simulink model "atrias_gear_dynamics"  (R2017a)
settings: Solver=ode45  StartTime=0.0  StopTime=sim_t  RelTol=1e-3  EnableMultiTasking=on
values from neighbouring files (symbols this model uses):
  N = grid_slice*1000    [createGrid.m]
  nm = fn_set_vnmc_params(sm, sample_time)    [kernel_scores_NM_mismatch.m]    (also in main_ATRIAS_cluster.m)
  nmc_BLCtrlPar = nmc.BLCtrlPar    [kernel_scores_NM_mismatch.m]    (also in main_ATRIAS_cluster.m)
  nmc_FPCtrlPar = nmc.FPCtrlPar    [kernel_scores_NM_mismatch.m]    (also in main_ATRIAS_cluster.m)
  nmc_LLCtrlPar = nmc.LLCtrlPar    [kernel_scores_NM_mismatch.m]    (also in main_ATRIAS_cluster.m)
  nmc_StCtrlPar = nmc.StCtrlPar    [kernel_scores_NM_mismatch.m]    (also in main_ATRIAS_cluster.m)
  nmc_SwCtrlPar = nmc.SwCtrlPar    [kernel_scores_NM_mismatch.m]    (also in main_ATRIAS_cluster.m)
  nmc_TrCtrlPar = nmc.TrCtrlPar    [kernel_scores_NM_mismatch.m]    (also in main_ATRIAS_cluster.m)
  nStep_switchCtrl = 10    [main_ATRIAS_cluster.m]
  nStep_thr = 1000    [createSimInitial.m]    (also in main_ATRIAS_cluster.m)
  rc_CtrlPar = [rc.k_placement, rc.T_step, rc.Cd, rc.kpt, rc.kdt, rc.desired_theta, rc.desired_z, rc.kpz, rc.kdz]    [kernel_scores_NM_mismatch.m]    (also in main_ATRIAS_cluster.m)
  sm = fn_set_MechParams(sm)    [kernel_scores_NM_mismatch.m]    (also in main_ATRIAS_cluster.m = fn_set_MechParams(sm,perturb))
  test_VNMC = 1    [createSimInitial.m]    (also in main_ATRIAS_cluster.m = 0)
undefined symbols (not defined in the file or in its folder): delta_phi_max, delta_phi_max_buffer, delta_phi_min, DiscIntNeverNeededParam, Discrete, idc, initial_dx_estimate, initial_dy_estimate, initial_dz_estimate, initial_z_estimate, kd_shin_max, kd_shin_min, kd_splay_max, kd_splay_min, kd_thigh_max, kd_thigh_min, kp_shin_max, kp_shin_min, kp_splay_max, kp_splay_min, kp_thigh_max, kp_thigh_min, mc, min_splay_angle, min_splay_buffer, phi_shin_max, phi_shin_max_buffer, phi_shin_min, phi_shin_min_buffer, phi_thigh_max, phi_thigh_max_buffer, phi_thigh_min, phi_thigh_min_buffer, rad, rc, s, sample_time, sgn, sim_d, t_friction, Time, X, Y, Z
libraries: sm_lib x206, nesl_utility x132, simulink x77, simulink_extras x24, mblibv1 x4, ctrlSharedLib x4, commnoisgen2 x1, dspswit3 x1
(part 17 of 17)

== stateflow chart atrias_gear_dynamics/control/Robot-to-NMM Interface/Contact State Machine1/State Machine ==
  state TouchDown
  state Unloading
  state Takeoff
  state Flight
  (junction 91) -> TouchDown
  TouchDown -> (junction 130) [order 2] : [vertical_grf < mc.contact_threshold]
  (junction 93) -> (junction 91)
  (junction 130) -> (junction 128)
  TouchDown -> Unloading [order 1] : [vertical_grf > mc.loaded_threshold]
  Unloading -> Takeoff : [vertical_grf < mc.contact_threshold]
  Takeoff -> Flight : after(rc.t_flight,sec)
  (default) -> Flight
  Flight -> (junction 93) : [vertical_grf > mc.contact_threshold]
  (junction 128) -> Flight
  data: z_velocity input; previous_z_velocity input; vertical_grf input; rc parameter; sm parameter; mc parameter; TouchDown output boolean; Unloading output boolean; Takeoff output boolean; Flight output boolean; vertical_acceleration input

== matlab function atrias_gear_dynamics/ATRIAS_sim/Mechanical System Layer/R Leg/Shin SEA/Rotor and Gearing Virtual approximate/gear dynamics approximate ==
  data: torque_rotor input; torque_load input; mc parameter; phi_l_dd output; phi_r_dd output; torque_torso output; gear_acc output; rotor_acc output
function [phi_l_dd, phi_r_dd, torque_torso, gear_acc, rotor_acc] = gear_dynamics_approx(torque_rotor, torque_load, mc)

% theta is the torso angle
% phi_r is the rotor local angle
% phi_l is the load local angle

N = mc.LEG_MTR_GEAR_RATIO;
It = mc.i_robot;
% It = It(2);
Ir = mc.j_rotor;
Il = mc.j_leg/N;

invM = [1/It 0 ; 0 1/(Ir*N^2)];
tau = [torque_rotor ; torque_load];
K = [-1 1 ; N 1];

out = invM*K*tau;

theta_dd = out(1);
torque_torso = It*theta_dd;

phi_l_dd = out(2) - out(1);
gear_acc = phi_l_dd;
phi_r_dd = N*phi_l_dd; 
rotor_acc = phi_r_dd;

% err = ((N-1)/It)*torque_rotor + (1/(N^2*Ir)+(N-1)^2/(N^2*It))*torque_load - out(2);

== matlab function atrias_gear_dynamics/ATRIAS_sim/Mechanical System Layer/R Leg/Thigh SEA/Rotor and Gearing Virtual approximate/gear dynamics approximate ==
  data: torque_rotor input; torque_load input; mc parameter; phi_l_dd output; phi_r_dd output; torque_torso output; gear_acc output; rotor_acc output
function [phi_l_dd, phi_r_dd, torque_torso, gear_acc, rotor_acc] = gear_dynamics_approx(torque_rotor, torque_load, mc)

% theta is the torso angle
% phi_r is the rotor local angle
% phi_l is the load local angle

N = mc.LEG_MTR_GEAR_RATIO;
It = mc.i_robot;
% It = It(2);
Ir = mc.j_rotor;
Il = mc.j_leg/N;

invM = [1/It 0 ; 0 1/(Ir*N^2)];
tau = [torque_rotor ; torque_load];
K = [-1 1 ; N 1];

out = invM*K*tau;

theta_dd = out(1);
torque_torso = It*theta_dd;

phi_l_dd = out(2) - out(1);
gear_acc = phi_l_dd;
phi_r_dd = N*phi_l_dd; 
rotor_acc = phi_r_dd;

% err = ((N-1)/It)*torque_rotor + (1/(N^2*Ir)+(N-1)^2/(N^2*It))*torque_load - out(2);

== matlab function atrias_gear_dynamics/ATRIAS_sim/Mechanical System Layer/Torso/Rotation To Euler Angles ==
  data: R input; roll output; pitch output; yaw output
function  [roll, pitch, yaw] = rotation_to_euler(R)  
    
    persistent curyaw
    if isempty(curyaw)
        curyaw = 0;
    end

    newyaw = atan2( R(2,1), R(1,1));
    pitch  = atan2(-R(3,1), sqrt(R(3,2)^2+R(3,3)^2));
    roll   = atan2( R(3,2), R(3,3));
    curyaw = curyaw + mod(newyaw - curyaw + pi, 2*pi) - pi;
    yaw = curyaw;
    
end

== matlab function atrias_gear_dynamics/control/Virtual Neuromuscular Control/Torque Distribution/mech limit avoidance1/PD Joint Limit1/to hip_knee ==
  data: Rtau_back input; tau_pd_hip_knee output; Rtau_front input; Ltau_back input; Ltau_front input; kR input; kL input
function tau_pd_hip_knee = fcn(Rtau_back,Rtau_front,Ltau_back,Ltau_front,kR,kL)

J_inv_trans = [1,1,0,0;
               -((kR+1)/(2*kR)),-((kR-1)/(2*kR)),0,0;
               0,0,1,1;
               0,0,-((kL+1)/(2*kL)),-((kL-1)/(2*kL))];
           
tau_pd_hip_knee = J_inv_trans*[Rtau_back;
                               Rtau_front;
                               Ltau_back;
                               Ltau_front];

== matlab function atrias_gear_dynamics/control/RC control/Inverse Dynamics 2D/target_GRF_inverse_dynamics ==
  data: GRFx input; GRFz input; z output; theta input; phi input; l_leg input; w input; tau_rotor_f input; tau_rotor_b input; mc parameter
%% Inverse dynamics
% Inputs:  gamma, dgamma, theta, dtheta,  GRFx_des, GRFy_des
% Outputs: ddx,   ddy,    ddl,   ddgamma, ddtheta,  tau_sf,  tau_sb
function z = fcn(GRFx, GRFz, theta, phi, l_leg, w,...
                                  tau_rotor_f, tau_rotor_b, ...
                                  mc)
              
    % Parameters
    m      = mc.m_total_real;    % mass of system + boom
    Il     = mc.j_leg;             % inertia of leg
    It     = mc.i_robot;           % inertia of system3.
    d      = mc.d_vertical_com;             % distance from hip to system COM
    g1     = phi(1)+theta(1);   % global leg angle (after spring)
    dg1    = phi(2)+theta(2);
    th     = theta(1);          % global torso angle   
    dth    = theta(2);
    t_rf   = tau_rotor_f;       % torque applied at front rotor 
    t_rb   = tau_rotor_b;       % torque applied at back rotor
    N      = -mc.LEG_MTR_GEAR_RATIO;
    l      = l_leg(1);          % leg length
    dl     = l_leg(2);
    g = mc.g;
    m_leg = mc.m_leg;
    
    % Stance dynamics (P z = [h; -dJ*dq] + [J zeros(2,2)]^T F)
    %     J  = [1  0  sin(g1)     l*cos(g1)   -d*cos(th);
    %           0  1  cos(g1)    -l*sin(g1)    d*sin(th)];
    %       
    %     dJ = [0  0   dg1*cos(g1)    (-l*dg1*sin(g1)+dl*cos(g1))  d*dth*sin(th);
    %           0  0  -dg1*sin(g1)    (-1*dg1*cos(g1)-dl*sin(g1))  d*dth*cos(th)];
    % 
    %     dq  = [dx  dz  dl  dg1  dth ]';
    %       
    %     M = [m  0   0       0    0; 
    %          0  m   0       0    0;
    %          0  0   m_leg   0    0;   
    %          0  0   0       Il   0;  
    %          0  0   0       0    It];  
    %     
    %     h = [0; -m*g_reduced; 0; 0; (-t_rf-t_rb)];
    % 
    %     S = [ 0         0;
    %           0         0;
    %           1/w      -1/w;
    %           1         1;
    %          -(N-1)/N  -(N-1)/N];
    % 
    %     F = [GRFx GRFz]';
    %     
    %     P = [M              -S;       
    %          J               zeros(2,2)];
    
    % Solving for z:    
    %     ddq = [ddx ddy ddl ddg1 ddth]';
    %     z = [ddq; t_sf; t_sb];
    %     z = P\([h; -dJ*dq] + [J zeros(2,2)]'*F);
    
    z =  [GRFx/m;
         (GRFz - g*m)/m;
        -(Il*d*dg1^2*m*cos(g1 - th) - 2*GRFx*Il*d*sin(th) - 2*Il*d^2*dth^2*m - GRFz*d*l^2*m*cos(th) - GRFx*d*l^2*m*sin(th) - 2*GRFz*Il*d*cos(th) + 2*GRFz*It*N*l*cos(g1) + 2*GRFz*Il*N*d*cos(th) + 2*GRFx*It*N*l*sin(g1) + 2*GRFx*Il*N*d*sin(th) - It*N*dg1^2*l*m + GRFz*d*l^2*m*cos(2*g1 - th) + GRFx*d*l^2*m*sin(2*g1 - th) + 2*Il*d*g*m*cos(th) + Il*d*dg1^2*m*cos(g1 + th) + 2*Il*N*d^2*dth^2*m - It*N*dg1^2*l^2*m - 2*It*N*g*l*m*cos(g1) - 2*Il*N*d*g*m*cos(th) + It*N*dg1^2*l^2*m*cos(2*g1) - Il*N*d*dg1^2*m*cos(g1 + th) - Il*d*dg1^2*l*m*cos(g1 + th) + 4*Il*d*dg1*dl*m*sin(g1 - th) + GRFz*N*d^2*l*m*cos(g1) + GRFz*N*d*l^2*m*cos(th) + GRFx*N*d^2*l*m*sin(g1) + 2*N*d*l*m*t_rb*sin(g1 - th) + 2*N*d*l*m*t_rf*sin(g1 - th) + GRFx*N*d*l^2*m*sin(th) - Il*N*d*dg1^2*m*cos(g1 - th) - GRFz*N*d^2*l*m*cos(g1 - 2*th) + GRFx*N*d^2*l*m*sin(g1 - 2*th) + Il*d*dg1^2*l*m*cos(g1 - th) - It*N*dg1^2*l*m*cos(2*g1) - GRFz*N*d*l^2*m*cos(2*g1 - th) - GRFx*N*d*l^2*m*sin(2*g1 - th) + Il*N*d*dg1^2*l*m*cos(g1 + th) - 4*Il*N*d*dg1*dl*m*sin(g1 - th) - Il*N*d*dg1^2*l*m*cos(g1 - th) + 2*It*N*d*dth^2*l*m*cos(g1 - th))/(2*m*(It*N*l - Il*d*cos(g1 - th) + Il*N*d*cos(g1 - th)));
        -(2*GRFx*It*N*cos(g1) - 2*GRFz*It*N*sin(g1) + GRFx*N*d^2*m*cos(g1 - 2*th) + 4*It*N*dg1*dl*m + GRFz*N*d^2*m*sin(g1 - 2*th) + GRFx*d*l*m*cos(2*g1 - th) - GRFz*d*l*m*sin(2*g1 - th) + It*N*dg1^2*m*sin(2*g1) + 2*It*N*g*m*sin(g1) + GRFx*d*l*m*cos(th) - GRFz*d*l*m*sin(th) + GRFx*N*d^2*m*cos(g1) + 2*N*d*m*t_rb*cos(g1 - th) + 2*N*d*m*t_rf*cos(g1 - th) - GRFz*N*d^2*m*sin(g1) - GRFx*N*d*l*m*cos(th) + GRFz*N*d*l*m*sin(th) - GRFx*N*d*l*m*cos(2*g1 - th) - 2*It*N*d*dth^2*m*sin(g1 - th) + GRFz*N*d*l*m*sin(2*g1 - th) - It*N*dg1^2*l*m*sin(2*g1))/(2*m*(It*N*l - Il*d*cos(g1 - th) + Il*N*d*cos(g1 - th)));
        -(GRFx*Il*cos(g1) - GRFz*Il*sin(g1) - GRFx*Il*N*cos(g1) + (Il*dg1^2*m*sin(2*g1))/2 + GRFz*Il*N*sin(g1) + Il*g*m*sin(g1) + GRFx*l^2*m*cos(g1) - GRFz*l^2*m*sin(g1) + 2*Il*dg1*dl*m + N*l*m*t_rb + N*l*m*t_rf + GRFz*N*l^2*m*sin(g1) - 2*Il*N*dg1*dl*m - Il*d*dth^2*m*sin(g1 - th) - (Il*N*dg1^2*m*sin(2*g1))/2 - (Il*dg1^2*l*m*sin(2*g1))/2 - Il*N*g*m*sin(g1) - GRFx*N*l^2*m*cos(g1) + GRFx*N*d*l*m*cos(th) - GRFz*N*d*l*m*sin(th) + Il*N*d*dth^2*m*sin(g1 - th) + (Il*N*dg1^2*l*m*sin(2*g1))/2)/(m*(It*N*l - Il*d*cos(g1 - th) + Il*N*d*cos(g1 - th)));
        -(2*GRFx*Il*It*N*cos(g1) - 2*GRFz*Il*It*N*sin(g1) - GRFz*Il*d*m*w*cos(th) - 2*GRFz*Il*d*m_leg*w*cos(th) - GRFx*Il*d*m*w*sin(th) - 2*GRFx*Il*d*m_leg*w*sin(th) + GRFx*Il*N*d^2*m*cos(g1) + 2*Il*N*d*m*t_rb*cos(g1 - th) + 2*Il*N*d*m*t_rf*cos(g1 - th) + 2*GRFx*It*N*l^2*m*cos(g1) - GRFz*Il*N*d^2*m*sin(g1) - 2*GRFz*It*N*l^2*m*sin(g1) + GRFx*Il*N*d^2*m*cos(g1 - 2*th) + 4*Il*It*N*dg1*dl*m + GRFz*Il*N*d^2*m*sin(g1 - 2*th) - 2*Il*d^2*dth^2*m*m_leg*w - GRFz*Il*d*m*w*cos(2*g1 - th) - GRFx*Il*d*m*w*sin(2*g1 - th) + Il*It*N*dg1^2*m*sin(2*g1) + 2*Il*It*N*g*m*sin(g1) - GRFx*d*l^2*m*m_leg*w*sin(th) - Il*It*N*dg1^2*l*m*sin(2*g1) + Il*d*dg1^2*m*m_leg*w*cos(g1 - th) + 2*GRFz*It*N*l*m*w*cos(g1) + 2*GRFz*It*N*l*m_leg*w*cos(g1) + GRFz*Il*N*d*m*w*cos(th) + 2*GRFz*Il*N*d*m_leg*w*cos(th) + 2*GRFx*It*N*l*m*w*sin(g1) + 2*GRFx*It*N*l*m_leg*w*sin(g1) + GRFx*Il*N*d*m*w*sin(th) + 2*GRFx*Il*N*d*m_leg*w*sin(th) - It*N*dg1^2*l*m*m_leg*w + GRFz*d*l^2*m*m_leg*w*cos(2*g1 - th) + GRFx*d*l^2*m*m_leg*w*sin(2*g1 - th) + 2*Il*d*g*m*m_leg*w*cos(th) + Il*d*dg1^2*m*m_leg*w*cos(g1 + th) + 2*Il*N*d^2*dth^2*m*m_leg*w - It*N*dg1^2*l^2*m*m_leg*w - 2*Il*It*N*d*dth^2*m*sin(g1 - th) + GRFz*Il*N*d*m*w*cos(2*g1 - th) + GRFx*Il*N*d*m*w*sin(2*g1 - th) - GRFz*d*l^2*m*m_leg*w*cos(th) + It*N*dg1^2*l^2*m*m_leg*w*cos(2*g1) - Il*N*d*dg1^2*m*m_leg*w*cos(g1 + th) - Il*d*dg1^2*l*m*m_leg*w*cos(g1 + th) + 4*Il*d*dg1*dl*m*m_leg*w*sin(g1 - th) + GRFz*N*d^2*l*m*m_leg*w*cos(g1) + GRFz*N*d*l^2*m*m_leg*w*cos(th) + GRFx*N*d^2*l*m*m_leg*w*sin(g1) + 2*N*d*l*m*m_leg*t_rb*w*sin(g1 - th) + 2*N*d*l*m*m_leg*t_rf*w*sin(g1 - th) + GRFx*N*d*l^2*m*m_leg*w*sin(th) - Il*N*d*dg1^2*m*m_leg*w*cos(g1 - th) - GRFz*N*d^2*l*m*m_leg*w*cos(g1 - 2*th) + GRFx*N*d^2*l*m*m_leg*w*sin(g1 - 2*th) + Il*d*dg1^2*l*m*m_leg*w*cos(g1 - th) - It*N*dg1^2*l*m*m_leg*w*cos(2*g1) - GRFz*N*d*l^2*m*m_leg*w*cos(2*g1 - th) - GRFx*N*d*l^2*m*m_leg*w*sin(2*g1 - th) - 2*It*N*g*l*m*m_leg*w*cos(g1) - 2*Il*N*d*g*m*m_leg*w*cos(th) + Il*N*d*dg1^2*l*m*m_leg*w*cos(g1 + th) - 4*Il*N*d*dg1*dl*m*m_leg*w*sin(g1 - th) - Il*N*d*dg1^2*l*m*m_leg*w*cos(g1 - th) + 2*It*N*d*dth^2*l*m*m_leg*w*cos(g1 - th))/(4*m*(It*N*l - Il*d*cos(g1 - th) + Il*N*d*cos(g1 - th)));
         (2*GRFz*Il*It*N*sin(g1) - 2*GRFx*Il*It*N*cos(g1) - GRFz*Il*d*m*w*cos(th) - 2*GRFz*Il*d*m_leg*w*cos(th) - GRFx*Il*d*m*w*sin(th) - 2*GRFx*Il*d*m_leg*w*sin(th) - GRFx*Il*N*d^2*m*cos(g1) - 2*Il*N*d*m*t_rb*cos(g1 - th) - 2*Il*N*d*m*t_rf*cos(g1 - th) - 2*GRFx*It*N*l^2*m*cos(g1) + GRFz*Il*N*d^2*m*sin(g1) + 2*GRFz*It*N*l^2*m*sin(g1) - GRFx*Il*N*d^2*m*cos(g1 - 2*th) - 4*Il*It*N*dg1*dl*m - GRFz*Il*N*d^2*m*sin(g1 - 2*th) - 2*Il*d^2*dth^2*m*m_leg*w - GRFz*Il*d*m*w*cos(2*g1 - th) - GRFx*Il*d*m*w*sin(2*g1 - th) - Il*It*N*dg1^2*m*sin(2*g1) - 2*Il*It*N*g*m*sin(g1) - GRFx*d*l^2*m*m_leg*w*sin(th) + Il*It*N*dg1^2*l*m*sin(2*g1) + Il*d*dg1^2*m*m_leg*w*cos(g1 - th) + 2*GRFz*It*N*l*m*w*cos(g1) + 2*GRFz*It*N*l*m_leg*w*cos(g1) + GRFz*Il*N*d*m*w*cos(th) + 2*GRFz*Il*N*d*m_leg*w*cos(th) + 2*GRFx*It*N*l*m*w*sin(g1) + 2*GRFx*It*N*l*m_leg*w*sin(g1) + GRFx*Il*N*d*m*w*sin(th) + 2*GRFx*Il*N*d*m_leg*w*sin(th) - It*N*dg1^2*l*m*m_leg*w + GRFz*d*l^2*m*m_leg*w*cos(2*g1 - th) + GRFx*d*l^2*m*m_leg*w*sin(2*g1 - th) + 2*Il*d*g*m*m_leg*w*cos(th) + Il*d*dg1^2*m*m_leg*w*cos(g1 + th) + 2*Il*N*d^2*dth^2*m*m_leg*w - It*N*dg1^2*l^2*m*m_leg*w + 2*Il*It*N*d*dth^2*m*sin(g1 - th) + GRFz*Il*N*d*m*w*cos(2*g1 - th) + GRFx*Il*N*d*m*w*sin(2*g1 - th) - GRFz*d*l^2*m*m_leg*w*cos(th) + It*N*dg1^2*l^2*m*m_leg*w*cos(2*g1) - Il*N*d*dg1^2*m*m_leg*w*cos(g1 + th) - Il*d*dg1^2*l*m*m_leg*w*cos(g1 + th) + 4*Il*d*dg1*dl*m*m_leg*w*sin(g1 - th) + GRFz*N*d^2*l*m*m_leg*w*cos(g1) + GRFz*N*d*l^2*m*m_leg*w*cos(th) + GRFx*N*d^2*l*m*m_leg*w*sin(g1) + 2*N*d*l*m*m_leg*t_rb*w*sin(g1 - th) + 2*N*d*l*m*m_leg*t_rf*w*sin(g1 - th) + GRFx*N*d*l^2*m*m_leg*w*sin(th) - Il*N*d*dg1^2*m*m_leg*w*cos(g1 - th) - GRFz*N*d^2*l*m*m_leg*w*cos(g1 - 2*th) + GRFx*N*d^2*l*m*m_leg*w*sin(g1 - 2*th) + Il*d*dg1^2*l*m*m_leg*w*cos(g1 - th) - It*N*dg1^2*l*m*m_leg*w*cos(2*g1) - GRFz*N*d*l^2*m*m_leg*w*cos(2*g1 - th) - GRFx*N*d*l^2*m*m_leg*w*sin(2*g1 - th) - 2*It*N*g*l*m*m_leg*w*cos(g1) - 2*Il*N*d*g*m*m_leg*w*cos(th) + Il*N*d*dg1^2*l*m*m_leg*w*cos(g1 + th) - 4*Il*N*d*dg1*dl*m*m_leg*w*sin(g1 - th) - Il*N*d*dg1^2*l*m*m_leg*w*cos(g1 - th) + 2*It*N*d*dth^2*l*m*m_leg*w*cos(g1 - th))/(4*m*(It*N*l - Il*d*cos(g1 - th) + Il*N*d*cos(g1 - th)))];


end

== matlab function atrias_gear_dynamics/control/RC control/Primary Secondary Leg Swap/ToggleRightLeftLeg ==
  data: toggle input boolean; right_left output double; previous_right_left input double; time_sim input
function right_left = ToggleRightLeftLeg(toggle, previous_right_left, time_sim)
    
    if toggle && time_sim > 0.1
        right_left = -previous_right_left + 1;
    else
        right_left = previous_right_left;
    end

end

== matlab function atrias_gear_dynamics/control/RC control/Sagittal State Feedback ==
  data: kpt input; kdt input; desired_theta input; Fx output size=1; x_dx input; z_dz input; theta_dtheta input; GRF_z input; idc parameter size=1; rc parameter
function Fx  = sagittal_feedback(kpt, kdt, desired_theta, x_dx, z_dz, theta_dtheta, GRF_z, idc, rc)
    sagittal_state = [x_dx(1),  x_dx(2), theta_dtheta(1), theta_dtheta(2)]';
    sagittal_reference = [0, 0 , desired_theta, 0]';
    sagittal_error = (sagittal_state - sagittal_reference);
    neutral_feedforward = GRF_z*x_dx(1)/z_dz(1);
    Fx_feedback =  -[rc.kpx, rc.kdx, kpt, kdt]*sagittal_error;
    Fx = Fx_feedback + neutral_feedforward;
    Fx = min(max(Fx,-0.5*GRF_z),0.5*GRF_z);
end

== matlab function atrias_gear_dynamics/control/RC control/Swing/swing_trajectory_regenerator ==
  data: T_step input; time_step input size=1; x output size=1; x0 input size=1; xd output size=1; xdd output size=1; z output size=1; zd output size=1; zdd output size=1; nstep input size=1; x1 input size=1; rc parameter size=1
function [x,xd,xdd, z,zd, zdd] = swing_trajectory_generator(T_step, time_step, x0, nstep, x1, rc)

%T_step = rc.T_step;
z_apex = rc.z_apex;

%x0 = -0.2;
dx0= 0.0;
% x1 = x1+0.05;
dx1 = 0.0;
z0 = 0.0;
dz0 = 0.0;
z1 = -0.05;
dz1 = 0.0;
T = T_step;

if(nstep == 1)
%     x0 = 0.0;
%     x1 = 0.2;
    z0 = 0.2;
    dz0 = 0.0;
    T = T_step/2;
end

tf = min(time_step, T);

if(tf < T/2)
    [a0 a1 a2 a3] = ThirdOrderTrajectory(z0, dz0, z_apex, 0.0, T/2);
    t = tf;
    z = a3*t^3 + a2*t^2 + a1*t + a0;
    zd = 3*a3*t^2 + 2*a2*t + a1;
else
    [a0 a1 a2 a3] = ThirdOrderTrajectory(z_apex, 0.0, z1, dz1, T/2);
    t = tf - T/2;
    z = a3*t^3 + a2*t^2 + a1*t + a0;
    zd = 3*a3*t^2 + 2*a2*t + a1;
end

zdd = 0;

[a0 a1 a2 a3] = ThirdOrderTrajectory(x0, dx0, x1, dx1, T);
t = tf;
x = a3*t^3 + a2*t^2 + a1*t + a0;
xd = 3*a3*t^2 + 2*a2*t + a1;
xdd = 6*a3*t + 2*a2;
end

== matlab function atrias_gear_dynamics/control/RC control/Torque Distribution/Motor Torque Saturation Optimization ==
  data: x1s input; t1 output; x2s input; mc parameter; t2 output
% Optimal leg motor torque distribution
function [t1, t2] = distribute_torque(x1s, x2s, mc)

lambda1 = mc.lambda1;
lambda2 = mc.lambda2;
max_torque_sagittal = mc.LEG_MTR_MAX_TORQUE;

s = max_torque_sagittal;

% possible solutions
x1 = [                                                      x1s;
                                                            0;
                                                            s;
                                                            0;
                                                           -s;
  (lambda2*s + lambda1*x1s - lambda2*x2s)/(lambda1 + lambda2);
  (lambda1*x1s - lambda2*s + lambda2*x2s)/(lambda1 + lambda2);
  (lambda2*s + lambda1*x1s + lambda2*x2s)/(lambda1 + lambda2);
 -(lambda2*s - lambda1*x1s + lambda2*x2s)/(lambda1 + lambda2)];
 
x2 = [                                                      x2s;
                                                            s;
                                                            0;
                                                           -s;
                                                            0;
  (lambda1*s - lambda1*x1s + lambda2*x2s)/(lambda1 + lambda2);
  (lambda1*s + lambda1*x1s + lambda2*x2s)/(lambda1 + lambda2);
  (lambda1*x1s - lambda1*s + lambda2*x2s)/(lambda1 + lambda2);
 -(lambda1*s + lambda1*x1s - lambda2*x2s)/(lambda1 + lambda2)];

% test constraints
c1 = s - x1 - x2 >= 0;
c2 = s + x1 + x2 >= 0;
c3 = s - x1 + x2 >= 0;
c4 = s + x1 - x2 >= 0;
constraints = c1 & c2 & c3 & c4;

% objective function to maximize
f = -lambda1*(x1-x1s).^2-lambda2*(x2-x2s).^2;
satisfied = find(constraints);
[~,I] = max(f(satisfied));

t1 = x1(satisfied(I));
t2 = x2(satisfied(I));

== matlab function atrias_gear_dynamics/control/RC control/Compute COM Translational Acceleration (IMU uses non-rotating measurement frame) ==
  data: com_acceleration_world output; torso_angular_accelerations input; imu_translational_accelerations_body input; torso_roll input; torso_pitch input; torso_yaw input; com_position_world input; com_velocity_world input; hip_roll_accelerations input; right_hip_roll input; left_hip_roll input; torso_com_acceleration_world output; pelvis_acceleration_world output; right_hip_acceleration_world output; left_hip_acceleration_world output; com_acceleration_yawed output; mc parameter
function [com_acceleration_world, torso_com_acceleration_world, pelvis_acceleration_world, right_hip_acceleration_world, left_hip_acceleration_world, com_acceleration_yawed] ...
          = compute_com_acceleration(torso_angular_accelerations, imu_translational_accelerations_body, torso_roll, torso_pitch, torso_yaw, ...
          com_position_world, com_velocity_world, ...
          hip_roll_accelerations, right_hip_roll, left_hip_roll, mc)

      pelvis_to_imu = mc.pelvis_to_imu;
      com_torso = mc.com_torso;
      com_leg_motor = mc.com_leg_motor;
      m_leg_motor = mc.m_leg_motor;
      m_leg = mc.m_leg;
      m_torso = mc.m_torso;
      g = mc.g;
      
    % Body frame to Yawed frame rotations  
    R_body_to_yawed = R_pitch(torso_pitch(1))*R_roll(torso_roll(1));
    dR_body_to_yawed = dR_pitch(torso_pitch(1),torso_pitch(2))*R_roll(torso_roll(1)) + R_pitch(torso_pitch(1))*dR_roll(torso_roll(1),torso_roll(2));
    ddR_body_to_yawed = ddR_pitch(torso_pitch(1),torso_pitch(2),torso_angular_accelerations(2))*R_roll(torso_roll(1)) ...
                        + R_pitch(torso_pitch(1))*ddR_roll(torso_roll(1),torso_roll(2),torso_angular_accelerations(1)) ... 
                        + 2*dR_pitch(torso_pitch(1),torso_pitch(2))*dR_roll(torso_roll(1),torso_roll(2));
    % Yawed frame to World frame rotations  
    R_yawed_to_world = R_yaw(torso_yaw(1));
    dR_yawed_to_world = dR_yaw(torso_yaw(1),torso_yaw(2));
    ddR_yawed_to_world = ddR_yaw(torso_yaw(1),torso_yaw(2),torso_angular_accelerations(3));
    % Compute translational acceleration of torso COM
    R_position_body_to_world = R_yawed_to_world*R_body_to_yawed;
    R_velocity_body_to_world = dR_yawed_to_world*R_body_to_yawed + R_yawed_to_world*dR_body_to_yawed;
    R_acceleration_body_to_world = ddR_yawed_to_world*R_body_to_yawed + 2*dR_yawed_to_world*dR_body_to_yawed + R_yawed_to_world*ddR_body_to_yawed;
    imu_to_torso_com_acceleration_world = R_acceleration_body_to_world*(com_torso - pelvis_to_imu)';
    imu_acceleration_world = R_yawed_to_world*R_body_to_yawed*imu_translational_accelerations_body;
    torso_com_acceleration_world = imu_acceleration_world + imu_to_torso_com_acceleration_world;
    % Compute accelerations of hip COMs
    R_right_hip_to_body =     R_roll(-pi/2+right_hip_roll(1));
    dR_right_hip_to_body =   dR_roll(-pi/2+right_hip_roll(1), right_hip_roll(2));
    ddR_right_hip_to_body = ddR_roll(-pi/2+right_hip_roll(1), right_hip_roll(2), hip_roll_accelerations(1));
    R_left_hip_to_body =     R_roll(pi/2-left_hip_roll(1));
    dR_left_hip_to_body =   dR_roll(pi/2-left_hip_roll(1), -left_hip_roll(2));
    ddR_left_hip_to_body = ddR_roll(pi/2-left_hip_roll(1), -left_hip_roll(2), -hip_roll_accelerations(2));
    imu_to_pelvis_com_acceleration_world = R_acceleration_body_to_world*(-pelvis_to_imu)';  
    pelvis_acceleration_world = imu_acceleration_world + imu_to_pelvis_com_acceleration_world;
    left_hip_acceleration_world = pelvis_acceleration_world + (R_acceleration_body_to_world*R_left_hip_to_body + 2*R_velocity_body_to_world*dR_left_hip_to_body + R_position_body_to_world*ddR_left_hip_to_body)*com_leg_motor';
    right_hip_acceleration_world = pelvis_acceleration_world + (R_acceleration_body_to_world*R_right_hip_to_body + 2*R_velocity_body_to_world*dR_right_hip_to_body + R_position_body_to_world*ddR_right_hip_to_body)*(com_leg_motor.*[1,-1,1])';
    % Compute total system COM acceleration
    m_hip = m_leg+m_leg_motor;
    m_total = 2*m_hip + m_torso;
    com_acceleration_world = (m_torso*torso_com_acceleration_world + m_hip*(left_hip_acceleration_world + right_hip_acceleration_world))/m_total;
    com_acceleration_yawed = ddR_yawed_to_world'*com_position_world + 2*dR_yawed_to_world'*com_velocity_world + R_yawed_to_world'*com_acceleration_world;
    com_acceleration_yawed(3) = com_acceleration_yawed(3);% - g;
end

function R_yp = R_pitch(theta) % map from pitched to yawed
  R_yp = [cos(theta), 0, sin(theta); ...
          0, 1, 0; ...
          -sin(theta), 0, cos(theta)];
end
function dR_yp = dR_pitch(theta,dtheta)
  dR_yp = dtheta*[-sin(theta), 0, cos(theta); ...
                  0, 0, 0; ... 
                  -cos(theta), 0, -sin(theta)];
end
function ddR_yp = ddR_pitch(theta,dtheta,ddtheta)
  ddR_yp = ddtheta*[-sin(theta), 0, cos(theta); ...
                    0, 0, 0; ... 
                    -cos(theta), 0, -sin(theta)] ...
           + dtheta^2*[-cos(theta), 0, -sin(theta); ...
                     0, 0, 0; ...
                     sin(theta), 0, -cos(theta)];
end
function R_pr = R_roll(phi) % map from rolled to pitched
  R_pr = [1, 0, 0; ...
          0, cos(phi), -sin(phi); ...
          0, sin(phi), cos(phi)]; 
end
function dR_pr = dR_roll(phi,dphi)
  dR_pr = dphi*[0, 0, 0; ...
                0, -sin(phi), -cos(phi); ...
                0, cos(phi), -sin(phi)];
end
function ddR_pr = ddR_roll(phi, dphi, ddphi)
  ddR_pr = ddphi*[0, 0, 0; ...
                  0, -sin(phi), -cos(phi); ...
                  0, cos(phi), -sin(phi)] ...
           + dphi^2*[0, 0, 0; ...
                   0, -cos(phi), sin(phi);...
                   0, -sin(phi), -cos(phi)];
end
function R_gy = R_yaw(psi) % map yawed frame to global
  R_gy = [cos(psi), -sin(psi), 0; sin(psi), cos(psi), 0; 0 0 1]; 
end
function dR_gy = dR_yaw(psi,dpsi)
  dR_gy = dpsi*[-sin(psi), -cos(psi), 0; cos(psi), -sin(psi), 0; 0 0 0];
end
function ddR_gy = ddR_yaw(psi,dpsi,ddpsi)
  ddR_gy = ddpsi*[-sin(psi), -cos(psi), 0; cos(psi), -sin(psi), 0; 0 0 0] ...
           + dpsi^2*[-cos(psi), sin(psi), 0; -sin(psi), -cos(psi), 0; 0 0 0];
end

== matlab function atrias_gear_dynamics/control/RC control/Compute World Frame COM Coordinates from Yawed Frame ==
  data: com_position_world output; X_dX input; Y_dY input; Z_dZ input; torso_yaw input; com_velocity_world output
function [com_position_world, com_velocity_world] ...
          = compute_com_state_in_world_frame(X_dX, Y_dY, Z_dZ, torso_yaw)

    R_yawed_to_world = R_yaw(torso_yaw(1));
    dR_yawed_to_world = dR_yaw(torso_yaw(1),torso_yaw(2));
    
    com_position_yawed = [X_dX(1); Y_dY(1); Z_dZ(1)];
    com_velocity_yawed = [X_dX(2); Y_dY(2); Z_dZ(2)];
    
    com_position_world = R_yawed_to_world*com_position_yawed;
    com_velocity_world = dR_yawed_to_world*com_position_yawed + R_yawed_to_world*com_velocity_yawed;

end

function R_gy = R_yaw(psi) % map yawed frame to global
  R_gy = [cos(psi), -sin(psi), 0; sin(psi), cos(psi), 0; 0 0 1]; 
end
function dR_gy = dR_yaw(psi,dpsi)
  dR_gy = dpsi*[-sin(psi), -cos(psi), 0; cos(psi), -sin(psi), 0; 0 0 0];
end

== matlab function atrias_gear_dynamics/control/Robot-to-NMM Interface/Force Estimation/Leg Force Measurements/Nonlinear Spring Force ==
  data: deflections input; tau_sea output
function tau_sea   = SeaSpringForce( deflections )
    tau_sea = SeaSpringForce( deflections );
end

== matlab function atrias_gear_dynamics/control/RC control/Atrias Swing control/Convert COM Position to Joint Angles + Leg Length  ==
  data: desired_leg_length output; X_star input; Y_star input; Z_star input; right_left input; com_pelvis_body input; desired_alpha output; desired_beta output; dcom_pelvis_body input; roll input; pitch input; sagittal_angle input; lateral_angle input; leg_length input; mc parameter
function [ desired_leg_length, desired_alpha, desired_beta ]  =  ...
          ConvertToJointAnglesAndLegLength(X_star, Y_star, Z_star, right_left,...
                           com_pelvis_body, dcom_pelvis_body, ...
                           roll, pitch, sagittal_angle, lateral_angle, leg_length,...
                           mc)
    lateral_offset = mc.lateral_offset;

    q = [roll(1), pitch(1), sagittal_angle(1), lateral_angle(1), leg_length(1)];
    dq = [roll(2), pitch(2), sagittal_angle(2), lateral_angle(2), leg_length(2)];
    [desired_alpha, desired_beta, desired_leg_length]  =  ConvertComPositionToLegAnglesAndLegLength(X_star, Y_star, Z_star, ~right_left, com_pelvis_body, dcom_pelvis_body, q, dq, lateral_offset);   

end

== matlab function atrias_gear_dynamics/control/RC control/Atrias Swing control/Avoid Hitting Mechanical Limits ==
  data: back_cmd output double; front_cmd output double; dback_cmd output double; dfront_cmd output double; ddback_cmd output double; ddfront_cmd output double; back_desired input; dback_desired input; ddback_desired input; front_desired input; dfront_desired input; ddfront_desired input; mc parameter
%% Avoid joint limits by ensuring we don't command velocities/accelerations that would push us into them when we are close to them.
function [back_cmd, front_cmd, dback_cmd, dfront_cmd, ddback_cmd, ddfront_cmd] ...
    = AvoidFourbarLimits(back_desired,dback_desired, ddback_desired, ...
          front_desired, dfront_desired, ddfront_desired, ...
          mc)
      min_front_bar_angle = mc.min_front_bar_angle;
      max_front_bar_angle = mc.max_front_bar_angle;
      min_back_bar_angle = mc.min_back_bar_angle;
      max_back_bar_angle = mc.max_back_bar_angle;
      
    [back_cmd, front_cmd, dback_cmd, dfront_cmd, ddback_cmd, ddfront_cmd] = AvoidFourbarLimits(back_desired,dback_desired, ddback_desired, front_desired, dfront_desired, ddfront_desired, min_front_bar_angle, max_front_bar_angle, min_back_bar_angle, max_back_bar_angle);
end

== matlab function atrias_gear_dynamics/control/RC control/Atrias Swing control/Virtual Leg to Four Bar ==
  data: l_leg input; dl_leg input; ddl_leg input; phi input; dphi input; ddphi input; back output; dback output; ddback output; front output; dfront output; ddfront output
 function [back, dback, ddback, front, dfront, ddfront] = VirtualLegToFourBar(l_leg, dl_leg, ddl_leg, phi, dphi, ddphi)
    [back, dback, ddback, front, dfront, ddfront] = VirtualLegToFourBar(l_leg, dl_leg, ddl_leg, phi, dphi, ddphi);
end

== matlab function atrias_gear_dynamics/control/RC control/lateralControl2D/2D Lateral Stance Control ==
  data: F_leg input; tau_primary output; desired_SecondaryLegRoll input; SecondaryLegRoll input; mc parameter; tau_secondary output; rc parameter
function [tau_primary, tau_secondary] = lateralControl2D(F_leg,desired_SecondaryLegRoll,SecondaryLegRoll,mc, rc)
    m_total_real = mc.m_total_real;
    m_leg_motor = mc.m_leg_motor;
    m_leg = mc.m_leg;
    k_lateral_swing_on_boom = rc.k_lateral_swing_on_boom;
    lateral_offset = mc.lateral_offset;
    
    tau_primary = F_leg*lateral_offset*(m_total_real-(m_leg_motor+m_leg))/m_total_real;
    tau_secondary = k_lateral_swing_on_boom'*([desired_SecondaryLegRoll(1); desired_SecondaryLegRoll(2)] - SecondaryLegRoll);
end

== matlab function atrias_gear_dynamics/control/RC control/State Estimation/Kalman Filtering/Measurement Noise Covariance Matricies ==
  data: R_no_position output; R_transverse output; vertical_GRF_L input; vertical_GRF_R input; mc parameter; sample_time parameter; R_vertical output; R_t_L output; R_t_R output
function [R_no_position, R_transverse, R_vertical, R_t_L,R_t_R] =...
         MeasurementNoiseCovariance(vertical_GRF_L, vertical_GRF_R, ...
           mc, sample_time)

    % filter states: [dx_w]; [dy_w]; [dz_w];
    % measurements:  [dx_w-dfL + dfL_hat; dx_w-dfR + dfR_hat]; 
    R_kalman_foot_stance = mc.R_kalman_foot_stance;
    R_kalman_foot_slip = mc.R_kalman_foot_slip;
    R_kalman_accelerometer = mc.R_kalman_accelerometer;
    R_kalman_dfoot_stance = mc.R_kalman_dfoot_stance;
    R_kalman_dfoot_slip = mc.R_kalman_dfoot_slip;
    m_total_real = mc.m_total_real;
    kalman_stance_slip_threshold = mc.kalman_stance_slip_threshold;
    g = mc.g;
    
    ratio_L = max(0, min(vertical_GRF_L/(kalman_stance_slip_threshold*m_total_real*g),1)); % ratio is 0 if no load, 1 if at least equilibrium
    ratio_R = max(0, min(vertical_GRF_R/(kalman_stance_slip_threshold*m_total_real*g),1));
    R_transverse = diag([ratio_L*R_kalman_foot_stance + (1-ratio_L)*R_kalman_foot_slip, ...
                         ratio_R*R_kalman_foot_stance + (1-ratio_R)*R_kalman_foot_slip, ...
                         R_kalman_accelerometer])/sample_time;
    R_vertical = diag([ratio_L*R_kalman_foot_stance  + (1-ratio_L)*R_kalman_foot_slip,...
                       ratio_R*R_kalman_foot_stance  + (1-ratio_R)*R_kalman_foot_slip,...
                       R_kalman_accelerometer])/sample_time;
                   
    R_no_position = diag([ratio_L*R_kalman_dfoot_stance + (1-ratio_L)*R_kalman_dfoot_slip, ...
                         ratio_R*R_kalman_dfoot_stance + (1-ratio_R)*R_kalman_dfoot_slip, ...
                         R_kalman_accelerometer])/sample_time;
                     
   R_t_L = R_transverse(1,1);
   R_t_R = R_transverse(2,2);
   
end

== matlab function atrias_gear_dynamics/control/RC control/State Estimation/Kalman Filtering/eigen values ==
  data: Z input; E output
function E = eigen(Z)
    E = real(eig(Z));
    E = sort(E);
end

== matlab function atrias_gear_dynamics/control/RC control/State Estimation/Kalman Filtering/eigen values1 ==
  data: Z input; E output
function E = eigen(Z)
    E = real(eig(Z));
    E = sort(E);
end

== matlab function atrias_gear_dynamics/control/RC control/State Estimation/Kalman Filtering/eigen values2 ==
  data: Z input; E output
function E = eigen(Z)
    E = real(eig(Z));
    E = sort(E);
end

== matlab function atrias_gear_dynamics/control/RC control/State Estimation/PositionUsingRobotGeometry ==
  data: com_left_foot output; dcom_left_foot output; com_right_foot output; dcom_right_foot output; right_left input; horizontal_com_position output; roll input; pitch input; yaw input; horizontal_com_velocity output; lateral_com_position output; lateral_com_velocity output; left_leg_sagittal_angle input; left_leg_lateral_angle input; left_leg_length input; right_leg_sagittal_angle input; right_leg_lateral_angle input; right_leg_length input; mc parameter; vertical_com_position output; vertical_com_velocity output; com_pelvis output; dcom_pelvis output
 % Returns 2D COM relative to primary foot
function [com_left_foot, dcom_left_foot, com_right_foot, dcom_right_foot,...
          horizontal_com_position, horizontal_com_velocity, ...
          lateral_com_position, lateral_com_velocity, ...
          vertical_com_position, vertical_com_velocity, ...
          com_pelvis, dcom_pelvis] = ...
         ComPositionUsingRobotGeometry(right_left, ...
                                    roll, pitch, yaw, ...
                                    left_leg_sagittal_angle, left_leg_lateral_angle, left_leg_length, ...
                                    right_leg_sagittal_angle, right_leg_lateral_angle, right_leg_length, ...
                                    mc)
                    

    m_torso = mc.m_torso;
    m_leg_motor = mc.m_leg_motor;
    m_leg = mc.m_leg;
    com_torso = mc.com_torso;
    com_leg_motor = mc.com_leg_motor;
    lateral_offset = mc.lateral_offset;
                                
    q =  [roll(1), pitch(1), yaw(1), left_leg_sagittal_angle(1), left_leg_lateral_angle(1), left_leg_length(1), right_leg_sagittal_angle(1), right_leg_lateral_angle(1), right_leg_length(1)];
    dq = [roll(2), pitch(2), yaw(2), left_leg_sagittal_angle(2), left_leg_lateral_angle(2), left_leg_length(2), right_leg_sagittal_angle(2), right_leg_lateral_angle(2), right_leg_length(2)];
                    
    [ com_pelvis, dcom_pelvis, ...
      com_left_foot, dcom_left_foot, ...
      com_right_foot, dcom_right_foot ] = ...
    ComCalculationFromRobot( q, dq, m_torso, m_leg_motor, m_leg, com_torso, com_leg_motor, lateral_offset );

    if right_left
        com_position = com_right_foot(4:6);
        com_velocity = dcom_right_foot(4:6);
    else
        com_position = com_left_foot(4:6);
        com_velocity = dcom_left_foot(4:6);
    end


    horizontal_com_position = com_position(1);
    horizontal_com_velocity = com_velocity(1);
    lateral_com_position = com_position(2);
    lateral_com_velocity = com_velocity(2);
    vertical_com_position = com_position(3);
    vertical_com_velocity = com_velocity(3);

end
